simulink model "heli_q8"  (R2014a)
settings: Solver=ode1  StartTime=0.0  StopTime=inf  FixedStep=0.002  RelTol=1e-3
PostLoadFcn:
  | qc_set_target_type(getConfigSet(bdroot, 'QUARC Default Target Configuration'));
values from neighbouring files (symbols this model uses):
  J_e = (m_c * l_c * l_c) + (2 * m_p * l_h * l_h)    (= 1.033536)    [init_heli.m]
  J_lambda = (m_c * l_c * l_c) + (2 * m_p * (l_h * l_h + l_p * l_p))    (= 1.077636)    [init_heli.m]
  J_p = 2 * m_p * l_p * l_p    (= 0.0441)    [init_heli.m]
  Joystick_gain_x = 1    [init_heli.m]
  Joystick_gain_y = -1    [init_heli.m]
  K_1 = L_1 / J_p    (= 0.619318181818)    [init_heli.m]
  K_2 = L_3 / J_e    (= 0.0996627113134)    [init_heli.m]
  K_3 = L_4 * V_s / J_lambda    (= -0.611739028763)    [init_heli.m]
  k_pd = sqrt(4 * k_pp / K_1)    [init_heli.m]
  k_pp = 4    [init_heli.m]
  k_rp = -1.5    [init_heli.m]
  L_1 = l_p * k_f    (= 0.0273119318182)    [init_heli.m]
  L_2 = (m_c * g * l_c) - (2 * m_p * g * l_h)    (= -0.659232)    [init_heli.m]
  L_3 = k_f * l_h    (= 0.103005)    [init_heli.m]
  L_4 = -k_f * l_h    (= -0.103005)    [init_heli.m]
  RadToDeg = 1/DegToRad    (= 57.2957795131)    [init_heli.m]
undefined symbols (not defined in the file or in its folder): HIL, qc_get_step_size
libraries: simulink_extras x6, quarc_library x4
settings Model: SimulationMode=external  ExtModeTrigDuration=5000  Creator=Rchan  LastModifiedBy=ernstt
settings SolverCC: PositivePriorityOrder=on
settings DataIOCC: SignalLoggingSaveFormat=ModelDataLogs
settings OptimizationCC: ExpressionDepthLimit=2147483647  InitFltsAndDblsToZero=on
settings DebuggingCC: SaveWithParameterizedLinksMsg=none  UnderspecifiedInitializationDetection=Classic  MultiTaskDSMMsg=warning  MultiTaskCondExecSysMsg=none  FcnCallInpInsideContextMsg=UseLocalSettings  StateNameClashWarn=warning
settings RTWCC: SystemTargetFile=quarc_win64.tlc  TemplateMakefile=quarc_default_tmf  Description=QUARC Win64 Target  ProcessScript=quarc_win64_make_rtw_hook
settings STFCustomTargetCC: CPPClassGenCompliant=on
settings GRTTargetCC: ParMdlRefBuildCompliant=off  CompOptLevelCompliant=off  CombineOutputUpdateFcns=off  MatFileLogging=off  GRTInterface=on  ExtMode=on  ExtModeMexFile=quarc_comm

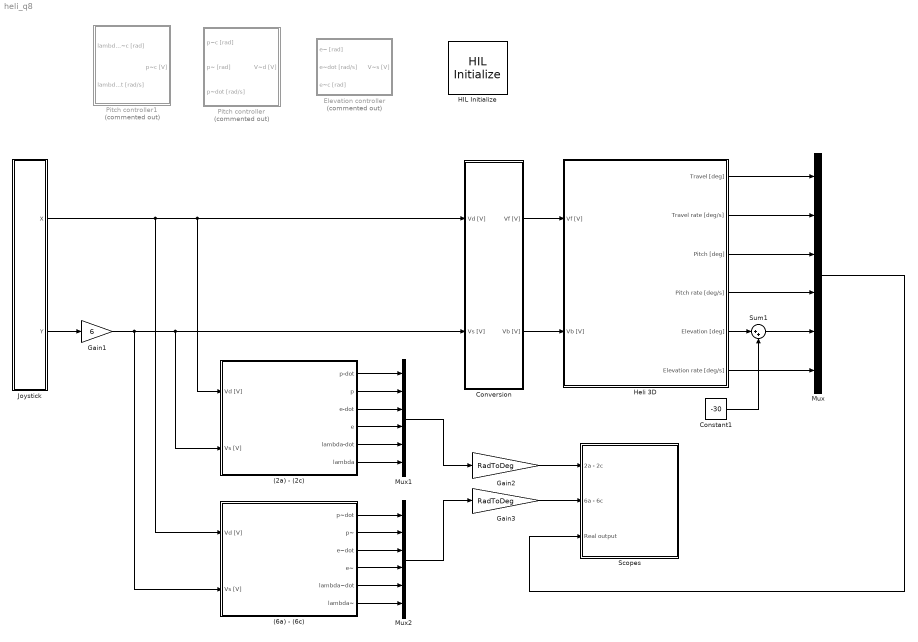
== system heli_q8 ==
  (2a) - (2c) : Subsystem
  (6a) - (6c) : Subsystem
  Constant1 : Constant  Value=-30
  Conversion : Subsystem
  Elevation controller : Subsystem  Commented=on
  Gain1 : Gain  Gain=6
  Gain2 : Gain  Gain=RadToDeg
  Gain3 : Gain  Gain=RadToDeg
  HIL Initialize : quarc_library/Data Acquisition/Generic/Configuration/HIL Initialize  Priority=-99  object_name=HIL-1  board_type=q8_usb  board_number=0  board_options=update_rate=normal;decimation=1  exclusive=off  active=off  hardware_clocks=[0:2]  clock_modes=[]  initial_clock_frequencies=[]  set_clock_params_at_start=off  set_clock_params_at_switch_in=off  set_clock_frequencies_at_start=off  set_clock_frequencies_at_switch_in=off  analog_input_channels=[0:7]  analog_input_maximums=10  analog_input_minimums=-10  set_analog_input_params_at_start=on  set_analog_input_params_at_switch_in=off  analog_output_channels=[0:7]  analog_output_maximums=10  analog_output_minimums=-10  initial_analog_outputs=[0]  final_analog_outputs=[0]  watchdog_analog_outputs=0  set_analog_output_params_at_start=on  set_analog_output_params_at_switch_in=off  set_analog_outputs_at_start=on  set_analog_outputs_at_switch_in=off  set_analog_outputs_at_terminate=on  set_analog_outputs_at_switch_out=off  set_analog_outputs_on_watchdog=off  digital_input_channels=[]  digital_output_channels=[]  digital_output_configuration=[]  initial_digital_outputs=[1]  final_digital_outputs=[1]  watchdog_digital_outputs=[1]  set_digital_output_params_at_start=off  set_digital_output_params_at_switch_in=off  set_digital_outputs_at_start=on  set_digital_outputs_at_switch_in=off  set_digital_outputs_at_terminate=on  set_digital_outputs_at_switch_out=off  set_digital_outputs_on_watchdog=off  encoder_channels=[0:7]  quadrature=[4]  encoder_filter_frequency=[]  initial_encoder_counts=[0]  set_encoder_params_at_start=on  set_encoder_params_at_switch_in=off  set_encoder_counts_at_start=on  set_encoder_counts_at_switch_in=off  pwm_channels=[0:7]  pwm_modes=0  pwm_frequency=99.532799999999995e6/4095  pwm_configuration=[0]  pwm_alignment=[0]  pwm_polarity=[1]  pwm_leading_deadband=[0]  pwm_trailing_deadband=[0]  initial_pwm_outputs=[0]  final_pwm_outputs=[0]  watchdog_pwm_outputs=[0]  set_pwm_params_at_start=on  set_pwm_params_at_switch_in=off  set_pwm_outputs_at_start=on  set_pwm_outputs_at_switch_in=off  set_pwm_outputs_at_terminate=on  set_pwm_outputs_at_switch_out=off  set_pwm_outputs_on_watchdog=off  other_output_channels=[]  initial_other_outputs=[]  final_other_outputs=[]  watchdog_other_outputs=[]  set_other_outputs_at_start=off  set_other_outputs_at_switch_in=off  set_other_outputs_at_terminate=off  set_other_outputs_at_switch_out=off  set_other_outputs_on_watchdog=off
  Heli 3D : Subsystem
  Joystick : Subsystem
  Mux : Mux  Inputs=6
  Mux1 : Mux  Inputs=6
  Mux2 : Mux  Inputs=6
  Pitch controller : Subsystem  Commented=on
  Pitch controller1 : Subsystem  Commented=on
  Scopes : Subsystem
  Sum1 : Sum  Inputs=|++
  wires:
  Conversion/2(Vb [V]) -> Heli 3D/2(Vb [V])
  Conversion/1(Vf [V]) -> Heli 3D/1(Vf [V])
  Joystick/2(Y) -> Gain1/1
  Heli 3D/5(Elevation [deg]) -> Sum1/1
  Constant1/1 -> Sum1/2
  Heli 3D/3(Pitch [deg]) -> Mux/3
  Sum1/1 -> Mux/5
  Heli 3D/2(Travel rate [deg/s]) -> Mux/2
  Heli 3D/4(Pitch rate [deg/s]) -> Mux/4
  Heli 3D/6(Elevation rate [deg/s]) -> Mux/6
  Heli 3D/1(Travel [deg]) -> Mux/1
  Joystick/1(X) -> (6a) - (6c)/1(Vd [V]), (2a) - (2c)/1(Vd [V]), Conversion/1(Vd [V])
  (2a) - (2c)/1(p-dot) -> Mux1/1
  (2a) - (2c)/2(p) -> Mux1/2
  (2a) - (2c)/3(e-dot) -> Mux1/3
  (2a) - (2c)/4(e) -> Mux1/4
  (2a) - (2c)/5(lambda-dot) -> Mux1/5
  (2a) - (2c)/6(lambda) -> Mux1/6
  (6a) - (6c)/1(p~dot) -> Mux2/1
  (6a) - (6c)/2(p~) -> Mux2/2
  (6a) - (6c)/3(e~dot) -> Mux2/3
  (6a) - (6c)/4(e~) -> Mux2/4
  (6a) - (6c)/5(lambda~dot) -> Mux2/5
  (6a) - (6c)/6(lambda~) -> Mux2/6
  Mux1/1 -> Gain2/1
  Mux2/1 -> Gain3/1
  Mux/1 -> Scopes/3(Real output)
  Gain1/1 -> (6a) - (6c)/2(Vs [V]), Conversion/2(Vs [V]), (2a) - (2c)/2(Vs [V])
  Gain2/1 -> Scopes/1(2a - 2c)
  Gain3/1 -> Scopes/2(6a - 6c)

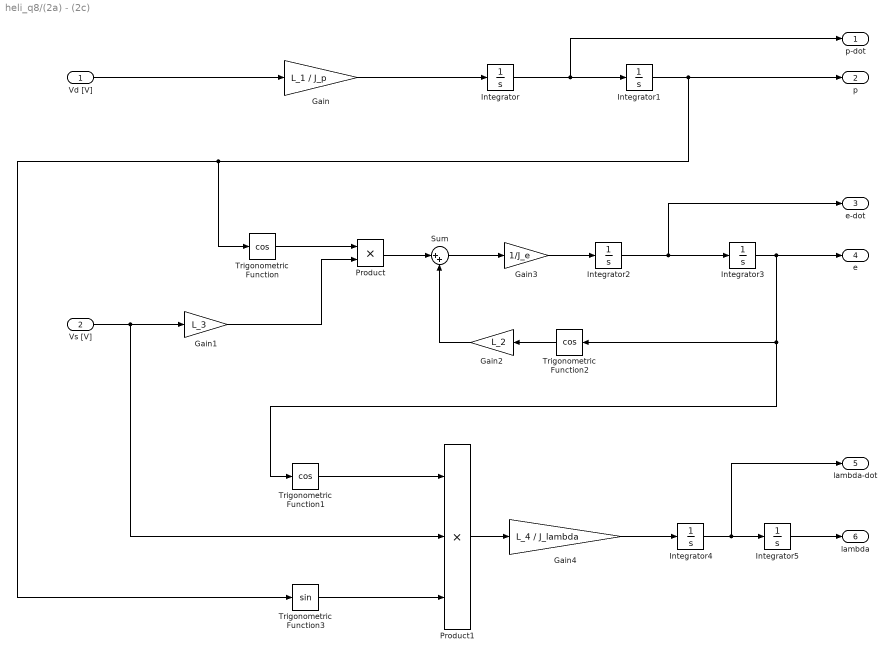
== system heli_q8/(2a) - (2c) ==
  Vd [V] : Inport
  Vs [V] : Inport  Port=2
  Gain : Gain  Gain=L_1 / J_p
  Gain1 : Gain  Gain=L_3
  Gain2 : Gain  Gain=L_2
  Gain3 : Gain  Gain=1/J_e
  Gain4 : Gain  Gain=L_4 / J_lambda
  Integrator{,1..5} (6 alike) : Integrator
  Product : Product
  Product1 : Product  Inputs=3
  Sum : Sum  Inputs=|++
  Trigonometric Function : Trigonometry  Operator=cos
  Trigonometric Function1 : Trigonometry  Operator=cos
  Trigonometric Function2 : Trigonometry  Operator=cos
  Trigonometric Function3 : Trigonometry
  p-dot : Outport
  p : Outport  Port=2
  e-dot : Outport  Port=3
  e : Outport  Port=4
  lambda-dot : Outport  Port=5
  lambda : Outport  Port=6
  wires:
  Vd [V]/1 -> Gain/1
  Gain/1 -> Integrator/1
  Integrator/1 -> p-dot/1, Integrator1/1
  Integrator1/1 -> Trigonometric Function3/1, Trigonometric Function/1, p/1
  Trigonometric Function/1 -> Product/1
  Vs [V]/1 -> Product1/2, Gain1/1
  Gain1/1 -> Product/2
  Product/1 -> Sum/1
  Trigonometric Function2/1 -> Gain2/1
  Gain2/1 -> Sum/2
  Sum/1 -> Gain3/1
  Integrator2/1 -> e-dot/1, Integrator3/1
  Integrator3/1 -> Trigonometric Function1/1, Trigonometric Function2/1, e/1
  Gain3/1 -> Integrator2/1
  Trigonometric Function1/1 -> Product1/1
  Trigonometric Function3/1 -> Product1/3
  Product1/1 -> Gain4/1
  Gain4/1 -> Integrator4/1
  Integrator4/1 -> lambda-dot/1, Integrator5/1
  Integrator5/1 -> lambda/1

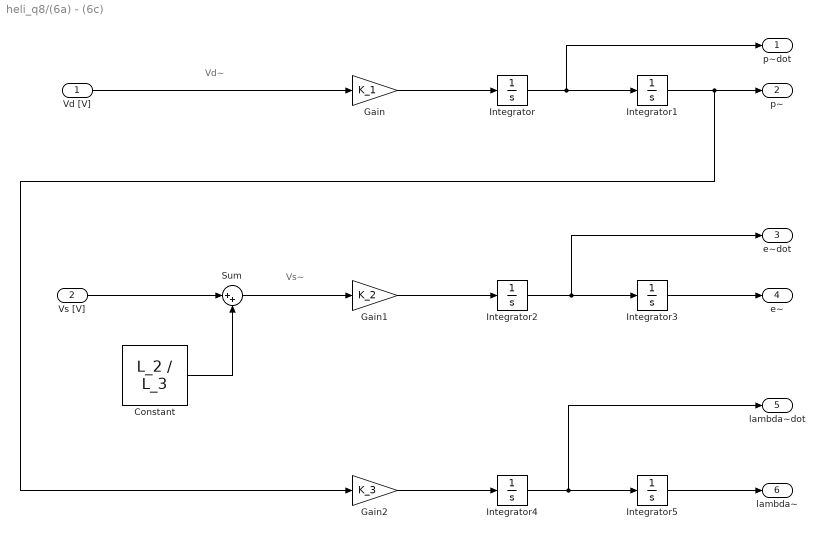
== system heli_q8/(6a) - (6c) ==
  note: Vs~
  note: Vd~
  Vd [V] : Inport
  Vs [V] : Inport  Port=2
  Constant : Constant  Value=L_2 / L_3
  Gain : Gain  Gain=K_1
  Gain1 : Gain  Gain=K_2
  Gain2 : Gain  Gain=K_3
  Integrator{,1..5} (6 alike) : Integrator
  Sum : Sum  Inputs=|++
  p~dot : Outport
  p~ : Outport  Port=2
  e~dot : Outport  Port=3
  e~ : Outport  Port=4
  lambda~dot : Outport  Port=5
  lambda~ : Outport  Port=6
  wires:
  Vd [V]/1 -> Gain/1
  Gain/1 -> Integrator/1
  Integrator/1 -> p~dot/1, Integrator1/1
  Integrator1/1 -> Gain2/1, p~/1
  Vs [V]/1 -> Sum/1
  Sum/1 -> Gain1/1
  Constant/1 -> Sum/2
  Gain1/1 -> Integrator2/1
  Integrator2/1 -> e~dot/1, Integrator3/1
  Integrator3/1 -> e~/1
  Integrator5/1 -> lambda~/1
  Integrator4/1 -> lambda~dot/1, Integrator5/1
  Gain2/1 -> Integrator4/1

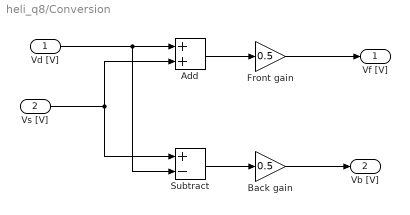
== system heli_q8/Conversion ==
  Vd [V] : Inport
  Vs [V] : Inport  Port=2
  Add : Sum
  Back gain : Gain  Gain=0.5
  Front gain : Gain  Gain=0.5
  Subtract : Sum  Inputs=+-
  Vf [V] : Outport
  Vb [V] : Outport  Port=2
  wires:
  Vd [V]/1 -> Subtract/2, Add/1
  Vs [V]/1 -> Subtract/1, Add/2
  Subtract/1 -> Back gain/1
  Back gain/1 -> Vb [V]/1
  Add/1 -> Front gain/1
  Front gain/1 -> Vf [V]/1

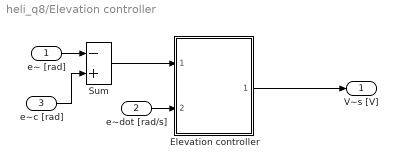
== system heli_q8/Elevation controller ==
  e~ [rad] : Inport
  e~dot [rad/s] : Inport  Port=2
  e~c [rad] : Inport  Port=3
  Elevation controller : Subsystem
  Sum : Sum  Inputs=-+  SaturateOnIntegerOverflow=on  InputSameDT=on  OutDataTypeStr=Inherit: Same as first input
  V~s [V] : Outport  InitialOutput=0
  wires:
  Sum/1 -> Elevation controller/1(e~ [rad])
  Elevation controller/1(V~_s [V]) -> V~s [V]/1
  e~ [rad]/1 -> Sum/1
  e~dot [rad/s]/1 -> Elevation controller/2(e~_dot [rad/s])
  e~c [rad]/1 -> Sum/2

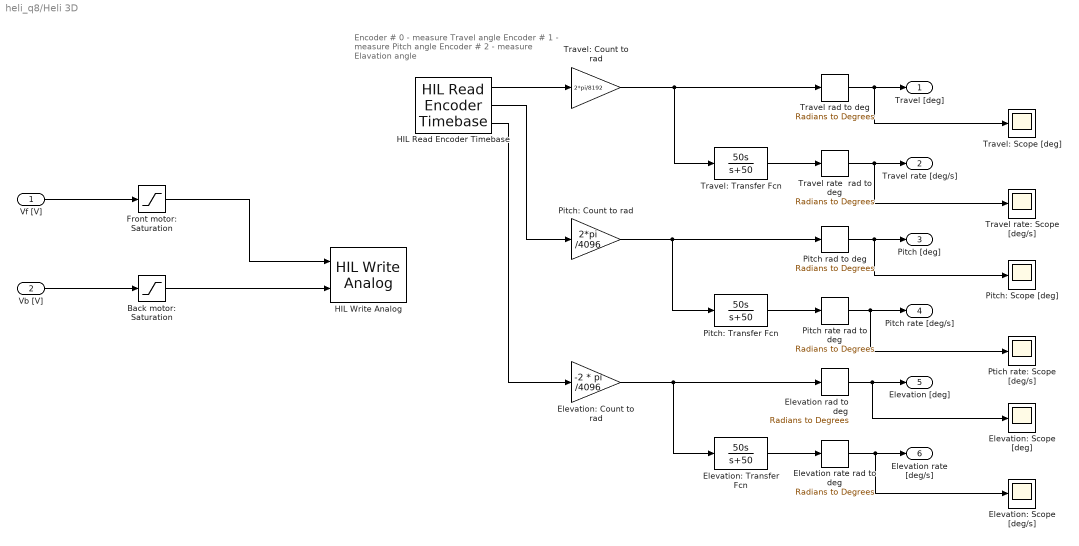
== system heli_q8/Heli 3D ==
  note: Encoder # 0 - measure Travel angle
      | Encoder # 1 - measure Pitch angle
      | Encoder # 2 - measure Elavation angle
  Vf [V] : Inport
  Vb [V] : Inport  Port=2
  Back motor: Saturation : Saturate  UpperLimit=5  LowerLimit=-5
  Elevation rad to deg : simulink_extras/Transformations/Radians to Degrees
  Elevation rate rad to deg : simulink_extras/Transformations/Radians to Degrees
  Elevation: Count to rad : Gain  Gain=-2 * pi /4096
  Elevation: Scope [deg/s] : Scope
      settings: YMin=-15  YMax=15  SaveName=ScopeData13
  Elevation: Scope [deg] : Scope
      settings: YMin=-15  YMax=15  SaveName=ScopeData12
  Elevation: Transfer Fcn : TransferFcn  Numerator=[50 0]  Denominator=[1 50]
  Front motor: Saturation : Saturate  UpperLimit=5  LowerLimit=-5
  HIL Read Encoder Timebase : quarc_library/Data Acquisition/Generic/Timebases/HIL Read Encoder Timebase  object_name=HIL-1  clock=0  channels=[0:2]  samples_in_buffer=max(ceil(1/qc_get_step_size), 1)  active=on  vector_output=off  data_type_mode=Inherit via back propagation  data_type=double
  HIL Write Analog : quarc_library/Data Acquisition/Generic/Immediate I//O/HIL Write Analog  object_name=HIL-1  channels=[0:1]  sample_time=-1  active=off  vector_input=off
  Pitch rad to deg : simulink_extras/Transformations/Radians to Degrees
  Pitch rate rad to deg : simulink_extras/Transformations/Radians to Degrees
  Pitch: Count to rad : Gain  Gain=2*pi /4096
  Pitch: Scope [deg] : Scope
      settings: YMin=-15  YMax=15  SaveName=ScopeData10
  Pitch: Transfer Fcn : TransferFcn  Numerator=[50 0]  Denominator=[1 50]
  Ptich rate: Scope [deg/s] : Scope
      settings: YMin=-15  YMax=15  SaveName=ScopeData11
  Travel rad to deg : simulink_extras/Transformations/Radians to Degrees
  Travel rate  rad to deg : simulink_extras/Transformations/Radians to Degrees
  Travel rate: Scope [deg/s] : Scope
      settings: YMin=-15  YMax=15  SaveName=ScopeData9
  Travel: Count to rad : Gain  Gain=2*pi/8192
  Travel: Scope [deg] : Scope
      settings: YMin=-15  YMax=15  SaveName=ScopeData8
  Travel: Transfer Fcn : TransferFcn  Numerator=[50 0]  Denominator=[1 50]
  Travel [deg] : Outport
  Travel rate [deg/s] : Outport  Port=2
  Pitch [deg] : Outport  Port=3
  Pitch rate [deg/s] : Outport  Port=4
  Elevation [deg] : Outport  Port=5
  Elevation rate [deg/s] : Outport  Port=6
  wires:
  HIL Read Encoder Timebase/1 -> Travel: Count to rad/1
  HIL Read Encoder Timebase/2 -> Pitch: Count to rad/1
  HIL Read Encoder Timebase/3 -> Elevation: Count to rad/1
  Travel: Count to rad/1 -> Travel: Transfer Fcn/1, Travel rad to deg/1
  Travel: Transfer Fcn/1 -> Travel rate  rad to deg/1
  Pitch: Count to rad/1 -> Pitch: Transfer Fcn/1, Pitch rad to deg/1
  Pitch: Transfer Fcn/1 -> Pitch rate rad to deg/1
  Elevation: Count to rad/1 -> Elevation: Transfer Fcn/1, Elevation rad to deg/1
  Elevation: Transfer Fcn/1 -> Elevation rate rad to deg/1
  Travel rad to deg/1 -> Travel: Scope [deg]/1, Travel [deg]/1
  Travel rate  rad to deg/1 -> Travel rate: Scope [deg/s]/1, Travel rate [deg/s]/1
  Pitch rad to deg/1 -> Pitch: Scope [deg]/1, Pitch [deg]/1
  Pitch rate rad to deg/1 -> Ptich rate: Scope [deg/s]/1, Pitch rate [deg/s]/1
  Elevation rad to deg/1 -> Elevation: Scope [deg]/1, Elevation [deg]/1
  Elevation rate rad to deg/1 -> Elevation: Scope [deg/s]/1, Elevation rate [deg/s]/1
  Vf [V]/1 -> Front motor: Saturation/1
  Vb [V]/1 -> Back motor: Saturation/1
  Front motor: Saturation/1 -> HIL Write Analog/1
  Back motor: Saturation/1 -> HIL Write Analog/2

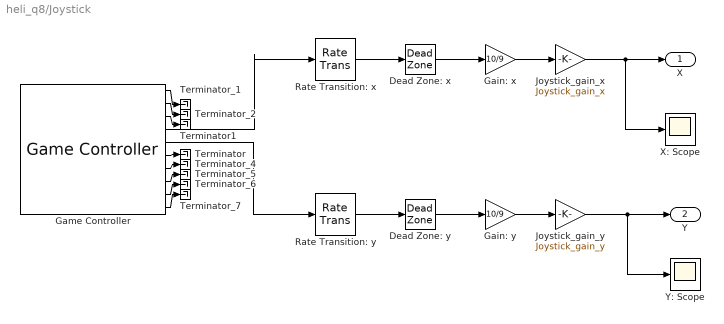
== system heli_q8/Joystick ==
  Dead Zone: x : DeadZone  LowerValue=-0.1  UpperValue=0.1  SaturateOnIntegerOverflow=on
  Dead Zone: y : DeadZone  LowerValue=-0.1  UpperValue=0.1  SaturateOnIntegerOverflow=on
  Gain: x : Gain  Gain=10/9
  Gain: y : Gain  Gain=10/9
  Game Controller : quarc_library/Devices/Peripherals/Target/Game Controller  controller=1  buffer_size=12  deadzone=[]  saturation=[]  sample_time=max(qc_get_step_size, 0.01)  auto_center=off  enabled=on
  Joystick_gain_x : Gain  Gain=Joystick_gain_x
  Joystick_gain_y : Gain  Gain=Joystick_gain_y
  Rate Transition: x : RateTransition
  Rate Transition: y : RateTransition
  Terminator : Terminator
  Terminator1 : Terminator
  Terminator_{1..2,4..7} (6 alike) : Terminator
  X: Scope : Scope
      settings: YMin=-1  YMax=1  SaveName=ScopeData7
  Y: Scope : Scope
      settings: YMin=-10  YMax=10  SaveName=ScopeData5
  X : Outport
  Y : Outport  Port=2
  wires:
  Rate Transition: y/1 -> Dead Zone: y/1
  Rate Transition: x/1 -> Dead Zone: x/1
  Game Controller/5 -> Rate Transition: y/1
  Game Controller/4 -> Rate Transition: x/1
  Game Controller/1 -> Terminator_1/1
  Game Controller/2 -> Terminator_2/1
  Game Controller/7 -> Terminator_4/1
  Game Controller/8 -> Terminator_5/1
  Game Controller/9 -> Terminator_6/1
  Game Controller/10 -> Terminator_7/1
  Game Controller/3 -> Terminator1/1
  Game Controller/6 -> Terminator/1
  Dead Zone: x/1 -> Gain: x/1
  Dead Zone: y/1 -> Gain: y/1
  Gain: x/1 -> Joystick_gain_x/1
  Gain: y/1 -> Joystick_gain_y/1
  Joystick_gain_x/1 -> X/1, X: Scope/1
  Joystick_gain_y/1 -> Y: Scope/1, Y/1

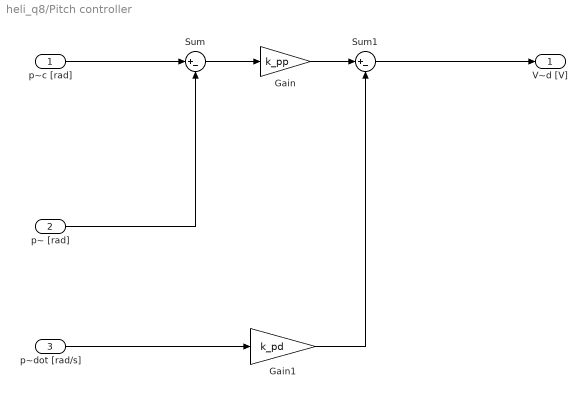
== system heli_q8/Pitch controller ==
  p~c [rad] : Inport
  p~ [rad] : Inport  Port=2
  p~dot [rad/s] : Inport  Port=3
  Gain : Gain  Gain=k_pp
  Gain1 : Gain  Gain=k_pd
  Sum : Sum  Inputs=|+-
  Sum1 : Sum  Inputs=|+-
  V~d [V] : Outport  InitialOutput=0
  wires:
  p~c [rad]/1 -> Sum/1
  p~ [rad]/1 -> Sum/2
  Sum/1 -> Gain/1
  Gain/1 -> Sum1/1
  p~dot [rad/s]/1 -> Gain1/1
  Gain1/1 -> Sum1/2
  Sum1/1 -> V~d [V]/1

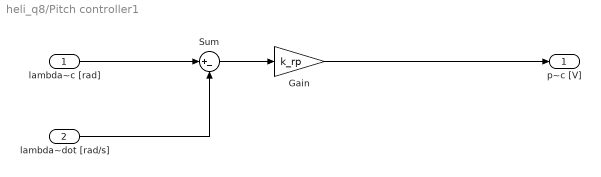
== system heli_q8/Pitch controller1 ==
  lambda~c [rad] : Inport
  lambda~dot [rad/s] : Inport  Port=2
  Gain : Gain  Gain=k_rp
  Sum : Sum  Inputs=|+-
  p~c [V] : Outport  InitialOutput=0
  wires:
  lambda~c [rad]/1 -> Sum/1
  Sum/1 -> Gain/1
  Gain/1 -> p~c [V]/1
  lambda~dot [rad/s]/1 -> Sum/2

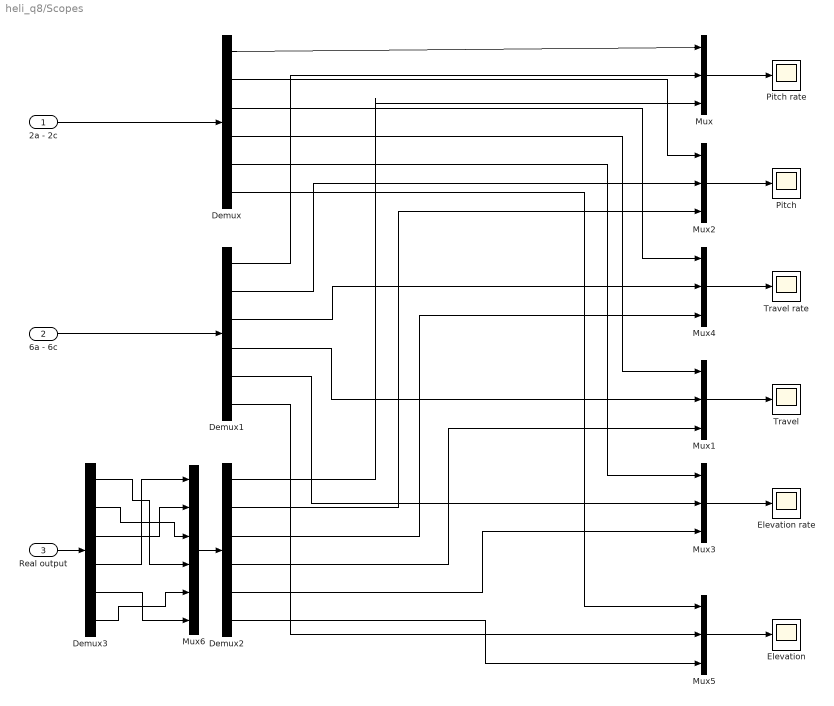
== system heli_q8/Scopes ==
  2a - 2c : Inport
  6a - 6c : Inport  Port=2
  Real output : Inport  Port=3
  Demux{,1..3} (4 alike) : Demux  Outputs=6
  "Elevation " : Scope
      settings: YMin=-4e+07  YMax=2.5e+06  SaveName=ScopeData6
  Elevation rate : Scope
      settings: YMin=-2.25  YMax=2.5  SaveName=ScopeData4
  Mux{,1..5} (6 alike) : Mux  Inputs=3
  Mux6 : Mux  Inputs=6
  "Pitch " : Scope
      settings: YMin=-2  YMax=1.5
  Pitch rate : Scope
      settings: YMin=-6  YMax=7
  "Travel " : Scope
      settings: YMin=-50000  YMax=2500  SaveName=ScopeData3
  Travel rate : Scope
      settings: YMin=-450  YMax=75  SaveName=ScopeData2
  wires:
  Mux/1 -> Pitch rate/1
  Mux2/1 -> "Pitch "/1
  Mux4/1 -> Travel rate/1
  Mux1/1 -> "Travel "/1
  Mux3/1 -> Elevation rate/1
  Mux5/1 -> "Elevation "/1
  6a - 6c/1 -> Demux1/1
  2a - 2c/1 -> Demux/1
  Demux/1 -> Mux/1
  Demux1/1 -> Mux/2
  Demux/2 -> Mux2/1
  Demux1/2 -> Mux2/2
  Demux/3 -> Mux4/1
  Demux1/3 -> Mux4/2
  Demux1/4 -> Mux1/2
  Demux/4 -> Mux1/1
  Demux/5 -> Mux3/1
  Demux/6 -> Mux5/1
  Demux1/5 -> Mux3/2
  Demux1/6 -> Mux5/2
  Real output/1 -> Demux3/1
  Mux6/1 -> Demux2/1
  Demux3/3 -> Mux6/2
  Demux3/4 -> Mux6/1
  Demux3/2 -> Mux6/3
  Demux3/1 -> Mux6/4
  Demux3/5 -> Mux6/6
  Demux3/6 -> Mux6/5
  Demux2/1 -> Mux/3
  Demux2/2 -> Mux2/3
  Demux2/3 -> Mux4/3
  Demux2/4 -> Mux1/3
  Demux2/5 -> Mux3/3
  Demux2/6 -> Mux5/3

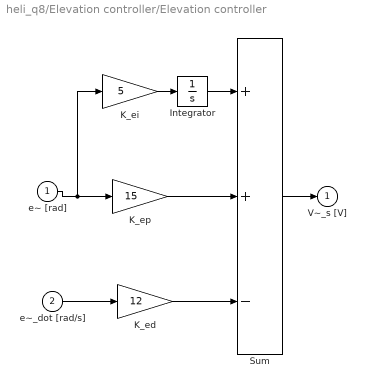
== system heli_q8/Elevation controller/Elevation controller ==
  e~ [rad] : Inport
  e~_dot [rad/s] : Inport  Port=2
  Integrator : Integrator  LimitOutput=on
  K_ed : Gain  Gain=12  SaturateOnIntegerOverflow=on  OutDataTypeStr=Inherit: Same as input  ParamDataTypeStr=Inherit: Same as input
  K_ei : Gain  Gain=5  SaturateOnIntegerOverflow=on  OutDataTypeStr=Inherit: Same as input  ParamDataTypeStr=Inherit: Same as input
  K_ep : Gain  Gain=15  SaturateOnIntegerOverflow=on  OutDataTypeStr=Inherit: Same as input  ParamDataTypeStr=Inherit: Same as input
  Sum : Sum  Inputs=++-  SaturateOnIntegerOverflow=on  InputSameDT=on  OutDataTypeStr=Inherit: Same as first input
  V~_s [V] : Outport  InitialOutput=0
  wires:
  K_ei/1 -> Integrator/1
  Integrator/1 -> Sum/1
  Sum/1 -> V~_s [V]/1
  e~_dot [rad/s]/1 -> K_ed/1
  K_ed/1 -> Sum/3
  K_ep/1 -> Sum/2
  e~ [rad]/1 -> K_ep/1, K_ei/1
